simulink model "integracao_condicional"  (R2023b)
settings: Solver=FixedStepAuto  StartTime=0.0  StopTime=50  FixedStep=parameters.ts  RelTol=1e-3
values from neighbouring files (symbols this model uses):
  parameters = back_calculation3(1)    [simulation1.m]    (also in simulation2.m = IntegracaoCondicional(1))
undefined symbols (not defined in the file or in its folder): DiscIntNeverNeededParam
libraries: simulink x1
settings Model: Creator=death  LastModifiedBy=nean

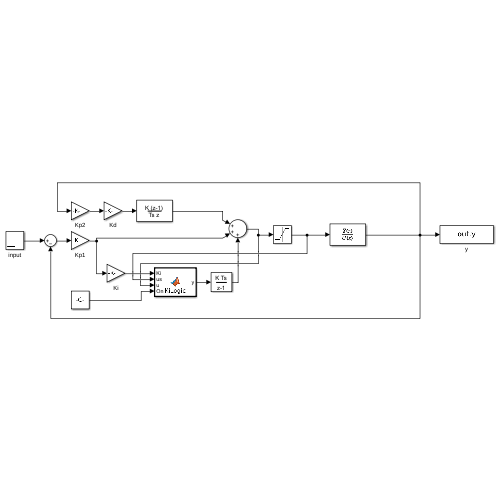
[thumbnail: Simulink's stored preview of the top-level diagram]
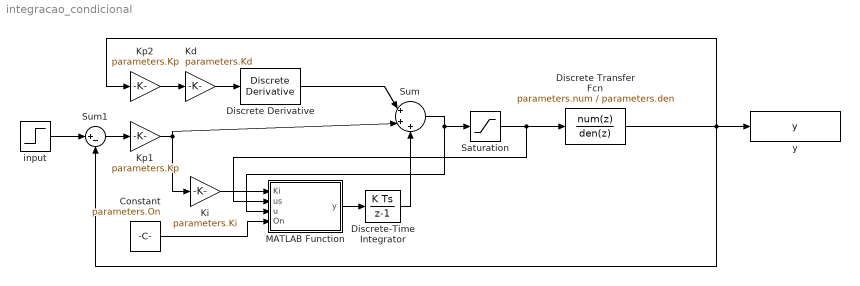
== system integracao_condicional ==
  Constant : Constant  Value=parameters.On
  Discrete Transfer Fcn : DiscreteTransferFcn  Numerator=parameters.num  Denominator=parameters.den
  Discrete Derivative : simulink/Discrete/Discrete Derivative  gainval=parameters.ts  ICPrevScaledInput=0.0  OutMin=[]  OutMax=[]  OutDataType=fixdt(1, 16)  OutScaling=2^-10  DoSatur=off
  Discrete-Time Integrator : DiscreteIntegrator  SampleTime=parameters.ts  ICPrevOutput=DiscIntNeverNeededParam  ICPrevScaledInput=DiscIntNeverNeededParam
  Kd : Gain  Gain=parameters.Kd
  Ki : Gain  Gain=parameters.Ki
  Kp1 : Gain  Gain=parameters.Kp
  Kp2 : Gain  Gain=parameters.Kp
  MATLAB Function : MATLAB Function  TreatAsAtomicUnit=on
  Saturation : Saturate  UpperLimit=parameters.upper_limit  LowerLimit=parameters.lower_limit
  Sum : Sum  Inputs=|+++
  Sum1 : Sum  Inputs=|+-
  input : Step  Time=parameters.step_time  Before=parameters.initial_value  After=parameters.final_value  SampleTime=parameters.sample_time
  y : ToWorkspace  VariableName=y  SaveFormat=Structure With Time  SampleTime=parameters.ts
  wires:
  Discrete Transfer Fcn/1 -> Sum1/2, y/1, Kp2/1
  Kp2/1 -> Kd/1
  Kd/1 -> Discrete Derivative/1
  Discrete-Time Integrator/1 -> Sum/3
  Discrete Derivative/1 -> Sum/1
  Kp1/1 -> Ki/1, Sum/2
  Sum1/1 -> Kp1/1
  Sum/1 -> MATLAB Function/3(u), Saturation/1
  input/1 -> Sum1/1
  MATLAB Function/1(y) -> Discrete-Time Integrator/1
  Ki/1 -> MATLAB Function/1(Ki)
  Saturation/1 -> MATLAB Function/2(us), Discrete Transfer Fcn/1
  Constant/1 -> MATLAB Function/4(On)

== matlab function integracao_condicional/MATLAB Function ==
  data: Ki input; y output; us input; u input; On input
function y = KiLogic(Ki, us, u, On)
    y = Ki;
    if (abs(u) > us && u > 0 && On == 1)
        y = 0;
    end
end
